simulink model "simACC"  (R2018a)
settings: Solver=VariableStepAuto  StartTime=0.0  StopTime=10.0  RelTol=1e-3
values from neighbouring files (symbols this model uses):
  c = 10    [ACC.m]
  ig = 6.267    [ACC.m]
  Ki = 2    [ACC.m]
  Kp = 10    [ACC.m]
  Kr = 3.0    (= 3)    [ACC.m]
  Kv = 1.5    [ACC.m]
  Kx = 40    [ACC.m]
  m = 400    [ACC.m]
  R0 = 2.0    (= 2)    [ACC.m]
  rw = 0.225    [ACC.m]
  Thw = 1.0    (= 1)    [ACC.m]
  tv = 0.2    [ACC.m]
libraries: simulink x1
settings Model: Creator=aoki-soya  LastModifiedBy=aoki-soya

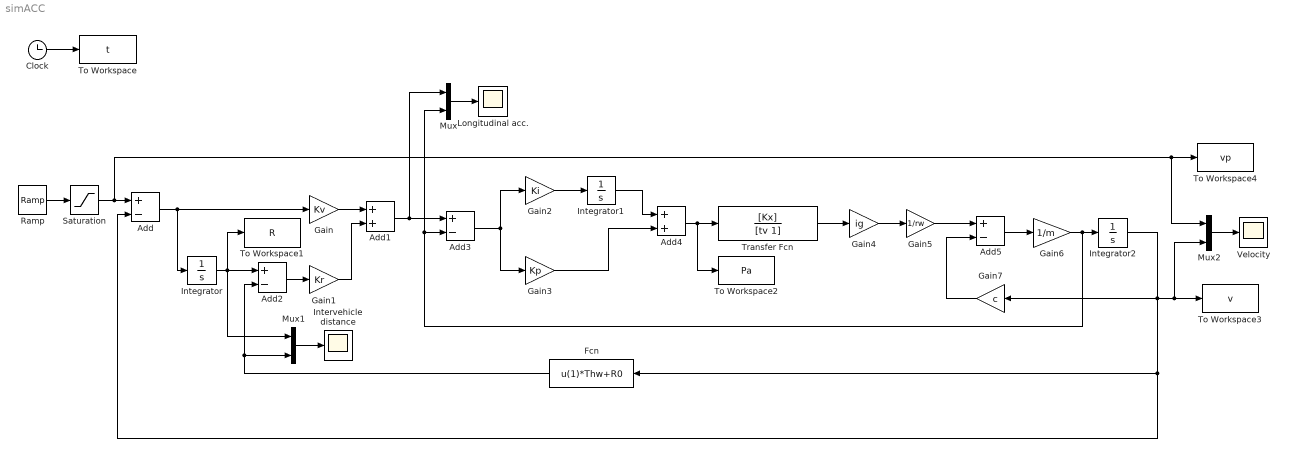
== system simACC ==
  Add{,2..3,5} (4 alike) : Sum  Inputs=+-
  Add1 : Sum
  Add4 : Sum
  Clock : Clock
      settings: Decimation=1/mydt
  Fcn : Fcn  Expr=u(1)*Thw+R0
  Gain : Gain  Gain=Kv
  Gain1 : Gain  Gain=Kr
  Gain2 : Gain  Gain=Ki
  Gain3 : Gain  Gain=Kp
  Gain4 : Gain  Gain=ig
  Gain5 : Gain  Gain=1/rw
  Gain6 : Gain  Gain=1/m
  Gain7 : Gain  Gain=c
  Integrator : Integrator  InitialCondition=R0
  Integrator1 : Integrator
  Integrator2 : Integrator  LimitOutput=on  LowerSaturationLimit=0
  Intervehicle distance : Scope
  Longitudinal acc. : Scope
  Mux : Mux  Inputs=2
  Mux1 : Mux  Inputs=2
  Mux2 : Mux  Inputs=2
  Ramp : simulink/Sources/Ramp  slope=1  start=0  InitialOutput=0
  Saturation : Saturate  UpperLimit=30/3.6  LowerLimit=0
  To Workspace : ToWorkspace  VariableName=t  SaveFormat=Timeseries  SampleTime=-1
  To Workspace1 : ToWorkspace  VariableName=R  SaveFormat=Timeseries  SampleTime=-1
  To Workspace2 : ToWorkspace  VariableName=Pa  SaveFormat=Timeseries  SampleTime=-1
  To Workspace3 : ToWorkspace  VariableName=v  SaveFormat=Timeseries  SampleTime=-1
  To Workspace4 : ToWorkspace  VariableName=vp  SaveFormat=Timeseries  SampleTime=-1
  Transfer Fcn : TransferFcn  Numerator=[Kx]  Denominator=[tv 1]
  Velocity : Scope
  wires:
  Ramp/1 -> Saturation/1
  Saturation/1 -> Mux2/1, To Workspace4/1, Add/1
  Add/1 -> Integrator/1, Gain/1
  Gain/1 -> Add1/1
  Integrator/1 -> Mux1/1, To Workspace1/1, Add2/1
  Add2/1 -> Gain1/1
  Gain1/1 -> Add1/2
  Add1/1 -> Add3/1, Mux/1
  Add3/1 -> Gain3/1, Gain2/1
  Gain2/1 -> Integrator1/1
  Integrator1/1 -> Add4/1
  Gain3/1 -> Add4/2
  Add4/1 -> To Workspace2/1, Transfer Fcn/1
  Transfer Fcn/1 -> Gain4/1
  Gain4/1 -> Gain5/1
  Gain5/1 -> Add5/1
  Add5/1 -> Gain6/1
  Gain6/1 -> Mux/2, Add3/2, Integrator2/1
  Gain7/1 -> Add5/2
  Fcn/1 -> Mux1/2, Add2/2
  Integrator2/1 -> Mux2/2, To Workspace3/1, Gain7/1, Add/2, Fcn/1
  Clock/1 -> To Workspace/1
  Mux/1 -> Longitudinal acc./1
  Mux1/1 -> Intervehicle distance/1
  Mux2/1 -> Velocity/1
